simulink library "thrust_estimation_v1"  (R2022a)
settings: Solver=VariableStepAuto  StartTime=0.0  StopTime=10.0  RelTol=1e-3
undefined symbols (not defined in the file): Config, DiscIntNeverNeededParam, Frames
libraries: WBToolboxLibrary x7, momentum_flight_control_sublib x1
settings Model: Creator=gnava  LastModifiedBy=gnava
settings SolverCC: AlgebraicLoopSolver=TrustRegion
settings DebuggingCC: UnconnectedInputMsg=warning  UnconnectedOutputMsg=warning  UnconnectedLineMsg=warning  SFMachineParentedDataDiag=warning
settings RTWCC: DLArmComputeVersion=19.05

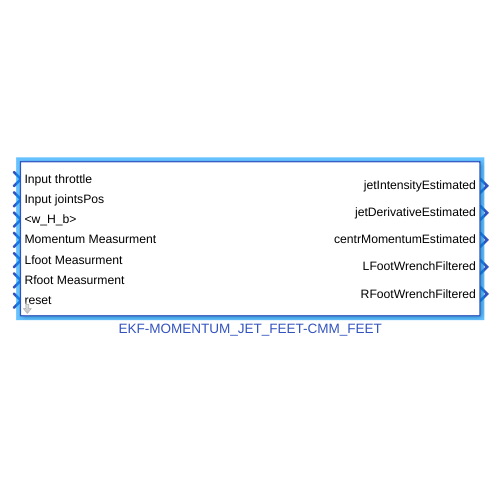
[thumbnail: Simulink's stored preview of the top-level diagram]
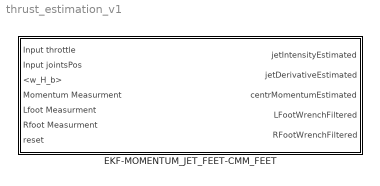
== system thrust_estimation_v1 ==
  EKF-MOMENTUM_JET_FEET-CMM_FEET : Subsystem  mask{Ts=Config.tStep, Frames=Frames, T0=[0.0; 0.0; 0.0; 0.0], dot_T0=[0.0; 0.0; 0.0; 0.0], h0=[0.0; 0.0; 0.0; 0.0; 0.0; 0.0], fLF0=[0.0; 0.0; 0.0; 0.0; 0.0; 0.0], fRF0=[0.0; 0.0; 0.0; 0.0; 0.0; 0.0], P0=blkdiag(eye(4)*1e1, eye(4)*1e1, eye(6)*1e1, eye(6)*1e1, eye(6)*1e1), Q=blkdiag(eye(4)*1e1, eye(4)*1e1, eye(6)*1e1, eye(6)*1e1, eye(6)*1e1), R=blkdiag(eye(6)*1e1, eye(6)*1e1, eye(6)*1e1), jetC_P100=Config.jetC_P100, jetC_P220=Config.jetC_P220}
      mask prompts: Ts "Sampling time Ts"; Frames "Frames Structure"; T0 "Initial Thrust T0"; dot_T0 "Initial Thrust Derivative dot_T0"; h0 "Initial Centroidal Momentum h_G0"; fLF0 "Initial Left Foot Contact Wrench"; fRF0 "Initial Right Foot Contact Wrench"; P0 "Initial Predicted covariance estimate"; Q "Process Covariance Matrix Q"; R "Meas. Covariance Matrix R"; jetC_P100 "P100 parameters"; jetC_P220 "P220 parameters"
      mask DialogControl Control2 Prompt: (Add text here)
      mask DialogControl Container4 Prompt: EKF Initial Values
      mask DialogControl Container5 Prompt: EKF noise assumptions
      mask DialogControl Container6 Prompt: Jets Parameters
      mask DialogControl Control3 Prompt: Further information about the block
      mask DialogControl Control4 Prompt: (Add text here and link in callback)
      mask DialogControl Control4 Callback: web https://github.com/dic-iit/element_ironcub-estimation/issues/48

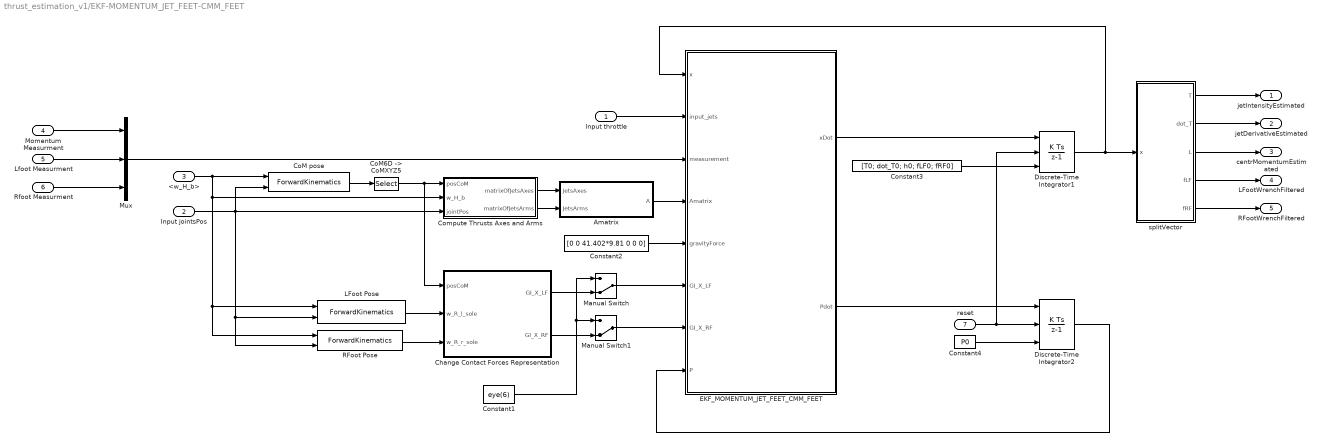
== system thrust_estimation_v1/EKF-MOMENTUM_JET_FEET-CMM_FEET ==
  Input throttle : Inport
  Input jointsPos : Inport  Port=2
  <w_H_b> : Inport  Port=3
  Momentum Measurment : Inport  Port=4
  Lfoot Measurment : Inport  Port=5
  Rfoot Measurment : Inport  Port=6
  reset : Inport  Port=7
  Amatrix : MATLAB Function  TreatAsAtomicUnit=on
  Change Contact Forces Representation : MATLAB Function  TreatAsAtomicUnit=on
  CoM pose : WBToolboxLibrary/Model/Kinematics/ForwardKinematics  frameName=Frames.COM_FRAME
      settings: SourceProductName=WholeBodyToolbox
  "CoM6D -> CoMXYZ5" : Selector  NumberOfDimensions=2  InputPortWidth=7  IndexOptions=Index vector (dialog),Index vector (dialog)  Indices=[1 2 3],[4]  OutputSizes=1,1
  Compute Thrusts Axes and Arms : Subsystem
  Constant1 : Constant  Value=eye(6)
  Constant2 : Constant  Value=[0 0 41.402*9.81 0 0 0]
  Constant3 : Constant  Value=[T0; dot_T0; h0; fLF0; fRF0]  VectorParams1D=off
  Constant4 : Constant  Value=P0
  Discrete-Time Integrator1 : DiscreteIntegrator  ExternalReset=rising  InitialConditionSource=external  SampleTime=Ts  ICPrevOutput=DiscIntNeverNeededParam  ICPrevScaledInput=DiscIntNeverNeededParam
  Discrete-Time Integrator2 : DiscreteIntegrator  ExternalReset=rising  InitialConditionSource=external  SampleTime=Ts  ICPrevOutput=DiscIntNeverNeededParam  ICPrevScaledInput=DiscIntNeverNeededParam
  "EKF_MOMENTUM_JET_FEET_CMM_FEET " : MATLAB Function  TreatAsAtomicUnit=on
  LFoot Pose : WBToolboxLibrary/Model/Kinematics/ForwardKinematics  frameName=Frames.LFOOT_FRAME
      settings: SourceProductName=WholeBodyToolbox
  Manual Switch : ManualSwitch  CurrentSetting=0
  Manual Switch1 : ManualSwitch  CurrentSetting=0
  Mux : Mux  Inputs=3
  RFoot Pose : WBToolboxLibrary/Model/Kinematics/ForwardKinematics  frameName=Frames.RFOOT_FRAME
      settings: SourceProductName=WholeBodyToolbox
  splitVector : MATLAB Function  TreatAsAtomicUnit=on
  jetIntensityEstimated : Outport  VectorParamsAs1DForOutWhenUnconnected=off
  jetDerivativeEstimated : Outport  Port=2  VectorParamsAs1DForOutWhenUnconnected=off
  centrMomentumEstimated : Outport  Port=3  VectorParamsAs1DForOutWhenUnconnected=off
  LFootWrenchFiltered : Outport  Port=4  VectorParamsAs1DForOutWhenUnconnected=off
  RFootWrenchFiltered : Outport  Port=5  VectorParamsAs1DForOutWhenUnconnected=off
  wires:
  Input throttle/1 -> "EKF_MOMENTUM_JET_FEET_CMM_FEET "/2(input_jets)
  Compute Thrusts Axes and Arms/2(matrixOfJetsArms) -> Amatrix/2(JetsArms)
  "EKF_MOMENTUM_JET_FEET_CMM_FEET "/1(xDot) -> Discrete-Time Integrator1/1
  Constant2/1 -> "EKF_MOMENTUM_JET_FEET_CMM_FEET "/5(gravityForce)
  "EKF_MOMENTUM_JET_FEET_CMM_FEET "/2(Pdot) -> Discrete-Time Integrator2/1
  Discrete-Time Integrator2/1 -> "EKF_MOMENTUM_JET_FEET_CMM_FEET "/8(P)
  Momentum Measurment/1 -> Mux/1
  Constant4/1 -> Discrete-Time Integrator2/3
  Constant3/1 -> Discrete-Time Integrator1/3
  CoM pose/1 -> "CoM6D -> CoMXYZ5"/1
  Discrete-Time Integrator1/1 -> "EKF_MOMENTUM_JET_FEET_CMM_FEET "/1(x), splitVector/1(x)
  Compute Thrusts Axes and Arms/1(matrixOfJetsAxes) -> Amatrix/1(JetsAxes)
  Amatrix/1(A) -> "EKF_MOMENTUM_JET_FEET_CMM_FEET "/4(Amatrix)
  <w_H_b>/1 -> RFoot Pose/1, LFoot Pose/1, Compute Thrusts Axes and Arms/2(w_H_b), CoM pose/1
  Manual Switch/1 -> "EKF_MOMENTUM_JET_FEET_CMM_FEET "/6(GI_X_LF)
  "CoM6D -> CoMXYZ5"/1 -> Change Contact Forces Representation/1(posCoM), Compute Thrusts Axes and Arms/1(posCoM)
  RFoot Pose/1 -> Change Contact Forces Representation/3(w_R_r_sole)
  Manual Switch1/1 -> "EKF_MOMENTUM_JET_FEET_CMM_FEET "/7(GI_X_RF)
  LFoot Pose/1 -> Change Contact Forces Representation/2(w_R_l_sole)
  Input jointsPos/1 -> CoM pose/2, RFoot Pose/2, LFoot Pose/2, Compute Thrusts Axes and Arms/3(jointPos)
  Rfoot Measurment/1 -> Mux/3
  Lfoot Measurment/1 -> Mux/2
  Mux/1 -> "EKF_MOMENTUM_JET_FEET_CMM_FEET "/3(measurement)
  splitVector/1(T) -> jetIntensityEstimated/1
  splitVector/5(fRF) -> RFootWrenchFiltered/1
  splitVector/4(fLF) -> LFootWrenchFiltered/1
  splitVector/3(L) -> centrMomentumEstimated/1
  splitVector/2(dot_T) -> jetDerivativeEstimated/1
  Constant1/1 -> Manual Switch1/1, Manual Switch/1
  Change Contact Forces Representation/1(GI_X_LF) -> Manual Switch/2
  Change Contact Forces Representation/2(GI_X_RF) -> Manual Switch1/2
  reset/1 -> Discrete-Time Integrator2/2, Discrete-Time Integrator1/2

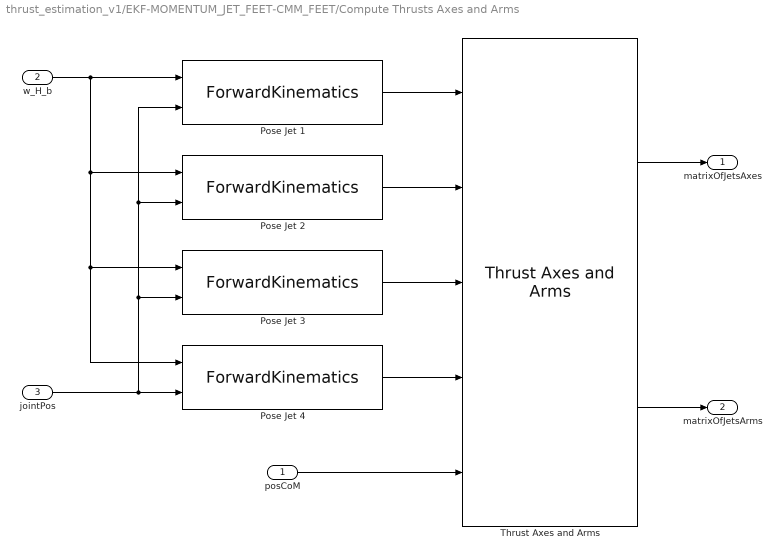
== system thrust_estimation_v1/EKF-MOMENTUM_JET_FEET-CMM_FEET/Compute Thrusts Axes and Arms ==
  posCoM : Inport
  w_H_b : Inport  Port=2
  jointPos : Inport  Port=3
  Pose Jet 1 : WBToolboxLibrary/Model/Kinematics/ForwardKinematics  frameName=Frames.JET1_FRAME
      settings: SourceProductName=WholeBodyToolbox
  Pose Jet 2 : WBToolboxLibrary/Model/Kinematics/ForwardKinematics  frameName=Frames.JET2_FRAME
      settings: SourceProductName=WholeBodyToolbox
  Pose Jet 3 : WBToolboxLibrary/Model/Kinematics/ForwardKinematics  frameName=Frames.JET3_FRAME
      settings: SourceProductName=WholeBodyToolbox
  Pose Jet 4 : WBToolboxLibrary/Model/Kinematics/ForwardKinematics  frameName=Frames.JET4_FRAME
      settings: SourceProductName=WholeBodyToolbox
  Thrust Axes and Arms : momentum_flight_control_sublib/Dynamics and Kinematics/Kinematic Quantities/Compute Thrusts Axes and Arms/Thrust Axes and Arms  SystemSampleTime=-1  VariantActivationTime=update diagram  Latency=0  AutoFrameSizeCalculation=off
      settings: SourceProductName=iRonCub Library
  matrixOfJetsAxes : Outport  VectorParamsAs1DForOutWhenUnconnected=off
  matrixOfJetsArms : Outport  Port=2  VectorParamsAs1DForOutWhenUnconnected=off
  wires:
  Pose Jet 2/1 -> Thrust Axes and Arms/2
  posCoM/1 -> Thrust Axes and Arms/5
  Thrust Axes and Arms/2 -> matrixOfJetsArms/1
  Thrust Axes and Arms/1 -> matrixOfJetsAxes/1
  Pose Jet 4/1 -> Thrust Axes and Arms/4
  Pose Jet 1/1 -> Thrust Axes and Arms/1
  Pose Jet 3/1 -> Thrust Axes and Arms/3
  w_H_b/1 -> Pose Jet 1/1, Pose Jet 2/1, Pose Jet 3/1, Pose Jet 4/1
  jointPos/1 -> Pose Jet 4/2, Pose Jet 3/2, Pose Jet 2/2, Pose Jet 1/2

== matlab function thrust_estimation_v1/EKF-MOMENTUM_JET_FEET-CMM_FEET/Amatrix ==
  data: JetsAxes input; JetsArms input; A output
function A  = AmatrixFCN(JetsAxes, JetsArms)

[A] = iRonCubLib.Amatrix(JetsAxes, JetsArms);

== matlab function thrust_estimation_v1/EKF-MOMENTUM_JET_FEET-CMM_FEET/EKF_MOMENTUM_JET_FEET_CMM_FEET  ==
  data: x input; input_jets input; measurement input; Amatrix input; gravityForce input; GI_X_LF input; GI_X_RF input; xDot output; P input; Q parameter; Pdot output; R parameter; jetC_P100 parameter; jetC_P220 parameter
function [xDot, Pdot] = EKF_MOMENTUM_JET_FEET_CMM_FEET_FNC(x, input_jets, measurement, Amatrix, gravityForce, GI_X_LF, GI_X_RF, P, Q, R, jetC_P100, jetC_P220)

[xDot, Pdot] = iRonCubLib.EKF_MOMENTUM_JET_FEET_CMM_FEET(x, input_jets,jetC_P100, jetC_P220, P, measurement, Amatrix, GI_X_LF, GI_X_RF, gravityForce, Q, R);

== matlab function thrust_estimation_v1/EKF-MOMENTUM_JET_FEET-CMM_FEET/splitVector ==
  data: x input; T output; dot_T output; L output; fLF output; fRF output
function [T, dot_T, L, fLF, fRF] = fcn(x)
T = x(1:4);
dot_T = x(5:8);
L = x(9:14);
fLF = x(15:20);
fRF = x(21:26);
end

== matlab function thrust_estimation_v1/EKF-MOMENTUM_JET_FEET-CMM_FEET/Change Contact Forces Representation ==
  data: posCoM input; GI_X_LF output; w_R_l_sole input; w_R_r_sole input; GI_X_RF output
function [GI_X_LF, GI_X_RF] = AdjWrenchTrBlockDiag(posCoM, w_R_l_sole, w_R_r_sole)

    % Distances between feet frames origins and the CoM position
    r_l_sole = w_R_l_sole(1:3,4) - posCoM;
    r_r_sole = w_R_r_sole(1:3,4) - posCoM;              

    % from body frame to mixed representation of the contact forces
    GI_X_LF = [w_R_l_sole(1:3,1:3),               zeros(3); ...
        wbc.skew(r_l_sole)*w_R_l_sole(1:3,1:3),   w_R_l_sole(1:3,1:3)];
    GI_X_RF = [w_R_r_sole(1:3,1:3),               zeros(3); ...
        wbc.skew(r_r_sole)*w_R_r_sole(1:3,1:3),   w_R_r_sole(1:3,1:3)];
end
